simulink model "Second_project"  (R2020a)
settings: Solver=VariableStepAuto  StartTime=0.0  StopTime=10.0  RelTol=1e-3
values from neighbouring files (symbols this model uses):
  x = input('Enter your Temperature in Celsius')    [script.m]
settings Model: Creator=mluser  LastModifiedBy=mluser

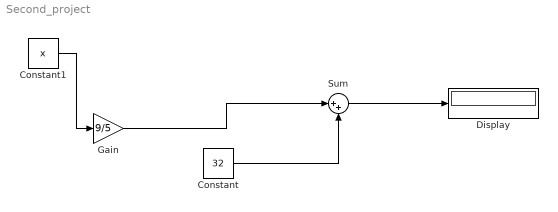
== system Second_project ==
  Constant : Constant  Value=32
  Constant1 : Constant  Value=x
  Display : Display
  Gain : Gain  Gain=9/5
  Sum : Sum  Inputs=|++
  wires:
  Constant/1 -> Sum/2
  Constant1/1 -> Gain/1
  Gain/1 -> Sum/1
  Sum/1 -> Display/1
